simulink model "CryoDet"  (R2015b)
settings: Solver=ode45  SolverMode=SingleTasking  StartTime=0.0  StopTime=1e-4  MaxStep=1e-9  RelTol=1e-3
values from neighbouring files (symbols this model uses):
  Fclk = Fadc    (= 307200000)    [setupCryoFPGAxray.m]
  freqBusAddrBits = 4    [setupCryoFPGAxray.m]
  noise = exp(2i*pi*rand(1, noiseLen))    [setupCryoFPGAxray.m]
  noiseLen = 128    [setupCryoFPGAxray.m]
  noiseSteps = 32    [setupCryoFPGAxray.m]
  Tclk = 1/Fclk    (= 3.25520833333e-09)    [setupCryoFPGAxray.m]
undefined symbols (not defined in the file or in its folder): AXI4, Lite, notch, notch2, notch3, notch4, xlipgetpartsetting
libraries: xbsIndex_r4 x1227
(part 4 of 9)

== system CryoDet/DspCore/AdcDac 0/twelveLineUDC 0 ==
  In1 : Inport
  BDC scope : Scope  NumInputPorts=2
  Constant : xbsIndex_r4/Constant  const=0  gui_display_data_type=Fixed-point  arith_type=Unsigned  n_bits=4  bin_pt=0  preci_type=Single  exp_width=8  frac_width=24  explicit_period=off  period=1  equ=P=C  opselect=C  inp2=PCIN>>17  opr=+  inp1=P  carry=CIN  dbl_ovrd=off  block_type=constant
  Constant1 : xbsIndex_r4/Constant  const=1  gui_display_data_type=Fixed-point  arith_type=Unsigned  n_bits=4  bin_pt=0  preci_type=Single  exp_width=8  frac_width=24  explicit_period=off  period=1  equ=P=C  opselect=C  inp2=PCIN>>17  opr=+  inp1=P  carry=CIN  dbl_ovrd=off  block_type=constant
  Constant10 : xbsIndex_r4/Constant  const=10  gui_display_data_type=Fixed-point  arith_type=Unsigned  n_bits=4  bin_pt=0  preci_type=Single  exp_width=8  frac_width=24  explicit_period=off  period=1  equ=P=C  opselect=C  inp2=PCIN>>17  opr=+  inp1=P  carry=CIN  dbl_ovrd=off  block_type=constant
  Constant11 : xbsIndex_r4/Constant  const=11  gui_display_data_type=Fixed-point  arith_type=Unsigned  n_bits=4  bin_pt=0  preci_type=Single  exp_width=8  frac_width=24  explicit_period=off  period=1  equ=P=C  opselect=C  inp2=PCIN>>17  opr=+  inp1=P  carry=CIN  dbl_ovrd=off  block_type=constant
  Constant12 : xbsIndex_r4/Constant  const=15  gui_display_data_type=Fixed-point  arith_type=Unsigned  n_bits=4  bin_pt=0  preci_type=Single  exp_width=8  frac_width=24  explicit_period=off  period=1  equ=P=C  opselect=C  inp2=PCIN>>17  opr=+  inp1=P  carry=CIN  dbl_ovrd=off  block_type=constant
  Constant2 : xbsIndex_r4/Constant  const=2  gui_display_data_type=Fixed-point  arith_type=Unsigned  n_bits=4  bin_pt=0  preci_type=Single  exp_width=8  frac_width=24  explicit_period=off  period=1  equ=P=C  opselect=C  inp2=PCIN>>17  opr=+  inp1=P  carry=CIN  dbl_ovrd=off  block_type=constant
  Constant3 : xbsIndex_r4/Constant  const=3  gui_display_data_type=Fixed-point  arith_type=Unsigned  n_bits=4  bin_pt=0  preci_type=Single  exp_width=8  frac_width=24  explicit_period=off  period=1  equ=P=C  opselect=C  inp2=PCIN>>17  opr=+  inp1=P  carry=CIN  dbl_ovrd=off  block_type=constant
  Constant4 : xbsIndex_r4/Constant  const=4  gui_display_data_type=Fixed-point  arith_type=Unsigned  n_bits=4  bin_pt=0  preci_type=Single  exp_width=8  frac_width=24  explicit_period=off  period=1  equ=P=C  opselect=C  inp2=PCIN>>17  opr=+  inp1=P  carry=CIN  dbl_ovrd=off  block_type=constant
  Constant5 : xbsIndex_r4/Constant  const=5  gui_display_data_type=Fixed-point  arith_type=Unsigned  n_bits=4  bin_pt=0  preci_type=Single  exp_width=8  frac_width=24  explicit_period=off  period=1  equ=P=C  opselect=C  inp2=PCIN>>17  opr=+  inp1=P  carry=CIN  dbl_ovrd=off  block_type=constant
  Constant6 : xbsIndex_r4/Constant  const=6  gui_display_data_type=Fixed-point  arith_type=Unsigned  n_bits=4  bin_pt=0  preci_type=Single  exp_width=8  frac_width=24  explicit_period=off  period=1  equ=P=C  opselect=C  inp2=PCIN>>17  opr=+  inp1=P  carry=CIN  dbl_ovrd=off  block_type=constant
  Constant7 : xbsIndex_r4/Constant  const=7  gui_display_data_type=Fixed-point  arith_type=Unsigned  n_bits=4  bin_pt=0  preci_type=Single  exp_width=8  frac_width=24  explicit_period=off  period=1  equ=P=C  opselect=C  inp2=PCIN>>17  opr=+  inp1=P  carry=CIN  dbl_ovrd=off  block_type=constant
  Constant8 : xbsIndex_r4/Constant  const=8  gui_display_data_type=Fixed-point  arith_type=Unsigned  n_bits=4  bin_pt=0  preci_type=Single  exp_width=8  frac_width=24  explicit_period=off  period=1  equ=P=C  opselect=C  inp2=PCIN>>17  opr=+  inp1=P  carry=CIN  dbl_ovrd=off  block_type=constant
  Constant9 : xbsIndex_r4/Constant  const=9  gui_display_data_type=Fixed-point  arith_type=Unsigned  n_bits=4  bin_pt=0  preci_type=Single  exp_width=8  frac_width=24  explicit_period=off  period=1  equ=P=C  opselect=C  inp2=PCIN>>17  opr=+  inp1=P  carry=CIN  dbl_ovrd=off  block_type=constant
  Counter : xbsIndex_r4/Counter  cnt_type=Count Limited  cnt_to=15  operation=Up  start_count=0  cnt_by_val=1  arith_type=Unsigned  n_bits=4  bin_pt=0  load_pin=off  rst=on  en=on  explicit_period=off  period=Tclk  use_behavioral_HDL=off  implementation=Fabric  dbl_ovrd=off  block_type=counter
  DAC Sum : Subsystem
  Delay : xbsIndex_r4/Delay  rst=off  infoeditControl=Selection of Reset will increase slice count due to use of real FFs and instead of SRLs  en=off  latency=6  reg_retiming=off  dbl_ovrd=off  block_type=delay
  Demux : Demux
  Gateway Out{1,7..10,23} (6 alike) : xbsIndex_r4/Gateway Out  inherit_from_input=off  hdl_port=off  rows=1  columns=1  UseAsDAC=off  DACChannel='1'  interface=None  automatic_assignment=on  address_offset=hex2dec('00')  intf_name=''  intf_description=''  timing_constraint=None  locs_specified=off  LOCs={}  io_standard={}  block_type=gatewayout
  Mux12X4 : Subsystem
  Mux6 : Mux  Inputs=2
  Mux7 : Mux  Inputs=2
  Relational : xbsIndex_r4/Relational  mode=a!=b  op_type=Bool  en=off  latency=0  dbl_ovrd=off  block_type=relational
  SBdemod : Subsystem
  Toolbar : xbsIndex_r4/Toolbar  func=xltoolbar  block_type=toolbar
      settings: infoedit=Toolbar
  oneLineUpDown0 : Subsystem
  oneLineUpDown1 : Subsystem
  oneLineUpDown10 : Subsystem
  oneLineUpDown11 : Subsystem
  oneLineUpDown2 : Subsystem
  oneLineUpDown3 : Subsystem
  oneLineUpDown4 : Subsystem
  oneLineUpDown5 : Subsystem
  oneLineUpDown6 : Subsystem
  oneLineUpDown7 : Subsystem
  oneLineUpDown8 : Subsystem
  oneLineUpDown9 : Subsystem
  synch scope : Scope  NumInputPorts=2
  toDAC : Outport
  demodulated : Outport  Port=2
  wires:
  [fpgaReset] -> Counter/1, Delay/1
  oneLineUpDown7/1(Out1) -> Mux12X4/8(line7)
  oneLineUpDown6/1(Out1) -> Mux12X4/7(line6)
  oneLineUpDown5/1(Out1) -> Mux12X4/6(line5)
  oneLineUpDown4/1(Out1) -> Mux12X4/5(line4)
  oneLineUpDown3/1(Out1) -> Mux12X4/4(line3)
  oneLineUpDown2/1(Out1) -> Mux12X4/3(line2)
  Mux12X4/1(Out1) -> SBdemod/1(In1)
  oneLineUpDown1/1(Out1) -> Mux12X4/2(line1)
  oneLineUpDown0/1(Out1) -> Mux12X4/1(line0)
  oneLineUpDown8/1(Out1) -> Mux12X4/9(line8)
  oneLineUpDown9/1(Out1) -> Mux12X4/10(line9)
  oneLineUpDown10/1(Out1) -> Mux12X4/11(line10)
  oneLineUpDown11/1(Out1) -> Mux12X4/12(line11)
  oneLineUpDown11/2(toDAC) -> DAC Sum/12(In12)
  oneLineUpDown10/2(toDAC) -> DAC Sum/11(In11)
  oneLineUpDown9/2(toDAC) -> DAC Sum/10(In10)
  oneLineUpDown8/2(toDAC) -> DAC Sum/9(In9)
  oneLineUpDown7/2(toDAC) -> DAC Sum/8(In8)
  oneLineUpDown6/2(toDAC) -> DAC Sum/7(In7)
  oneLineUpDown5/2(toDAC) -> DAC Sum/6(In6)
  oneLineUpDown4/2(toDAC) -> DAC Sum/5(In5)
  oneLineUpDown3/2(toDAC) -> DAC Sum/4(In4)
  oneLineUpDown2/2(toDAC) -> DAC Sum/3(In3)
  oneLineUpDown1/2(toDAC) -> DAC Sum/2(In2)
  oneLineUpDown0/2(toDAC) -> DAC Sum/1(In1)
  DAC Sum/1(Out1) -> toDAC/1
  SBdemod/1(AllComponents) -> demodulated/1
  Gateway Out10/1 -> Mux7/2
  Gateway Out9/1 -> Mux7/1
  Gateway Out8/1 -> Mux6/2
  Gateway Out7/1 -> Mux6/1
  Mux6/1 -> BDC scope/1
  Mux7/1 -> BDC scope/2
  Demux/1 -> Gateway Out7/1
  Demux/4 -> Gateway Out10/1
  Demux/3 -> Gateway Out9/1
  Demux/2 -> Gateway Out8/1
  Delay/1 -> Mux12X4/13(synch)
  Constant/1 -> oneLineUpDown0/2(addrIn)
  Constant1/1 -> oneLineUpDown1/2(addrIn)
  Constant2/1 -> oneLineUpDown2/2(addrIn)
  Constant3/1 -> oneLineUpDown3/2(addrIn)
  Constant4/1 -> oneLineUpDown4/2(addrIn)
  Constant5/1 -> oneLineUpDown5/2(addrIn)
  Constant6/1 -> oneLineUpDown6/2(addrIn)
  Constant7/1 -> oneLineUpDown7/2(addrIn)
  Constant8/1 -> oneLineUpDown8/2(addrIn)
  Constant9/1 -> oneLineUpDown9/2(addrIn)
  Constant10/1 -> oneLineUpDown10/2(addrIn)
  Constant11/1 -> oneLineUpDown11/2(addrIn)
  In1/1 -> oneLineUpDown6/1(In), oneLineUpDown8/1(In), oneLineUpDown9/1(In), oneLineUpDown10/1(In), oneLineUpDown11/1(In), oneLineUpDown7/1(In), Demux/1, oneLineUpDown5/1(In), oneLineUpDown4/1(In), oneLineUpDown3/1(In), oneLineUpDown2/1(In), oneLineUpDown1/1(In), oneLineUpDown0/1(In)
  Counter/1 -> Gateway Out23/1, Relational/2, oneLineUpDown2/3(synchIn), oneLineUpDown3/3(synchIn), oneLineUpDown4/3(synchIn), oneLineUpDown5/3(synchIn), oneLineUpDown6/3(synchIn), oneLineUpDown7/3(synchIn), oneLineUpDown8/3(synchIn), oneLineUpDown10/3(synchIn), oneLineUpDown11/3(synchIn), oneLineUpDown9/3(synchIn), oneLineUpDown1/3(synchIn), oneLineUpDown0/3(synchIn)
  Gateway Out23/1 -> synch scope/1
  Gateway Out1/1 -> synch scope/2
  Relational/1 -> Gateway Out1/1, Counter/2
  Constant12/1 -> Relational/1

== system CryoDet/DspCore/AdcDac 0/twelveLineUDC 1 ==
  note: Null for now, eventually copy twelveLineUDC 0
      | when we need more than 12 lines per ADC channel
  In1 : Inport
  Out1 : Outport
  wires:
  In1/1 -> Out1/1

== system CryoDet/DspCore/AdcDac 0/LPF/CIC reset ==
  note: where N is number of channels in CIC filter
  note: reset latched resetIn
  note: latch resetIn
  note: CIC reset
      |
      | Synchronizes a CIC compiler 4.0 multi-channel CIC filter
      | to input channels
      |
      | Generates:
      | 1	notResetOut to CIC aresetn
      | 2	tlast to CIC tlast input
      |
      | Inputs:
      | 1	reset in
      | 2	Channel number (0-N) which may go to sel input of mux generating the input data stream
      | 3	N-2 which tells this module how deep is the multiplexing (e.g. N-2 = 10 for a 12 channel CIC filter (sorry))
      |
      | Guarantees:
      | 1	reset out is at least 2 clocks long
      | 2	end of reset occurs 2 clocks before channel 0
      | 3	tlast comes with channel N-1
      |
      | Assumes:
      | CIC oversampling set to "Sample period" = 1
      | No "streaming interface"
  resetIn : Inport
  Channel : Inport  Port=2
  N-2 : Inport  Port=3
  Constant : xbsIndex_r4/Constant  const=0  gui_display_data_type=Boolean  arith_type=Boolean  n_bits=16  bin_pt=14  preci_type=Single  exp_width=8  frac_width=24  explicit_period=off  period=1  equ=P=C  opselect=C  inp2=PCIN>>17  opr=+  inp1=P  carry=CIN  dbl_ovrd=off  block_type=constant
  Delay1 : xbsIndex_r4/Delay  rst=off  infoeditControl=Selection of Reset will increase slice count due to use of real FFs and instead of SRLs  en=off  latency=1  reg_retiming=off  dbl_ovrd=off  block_type=delay
  Delay2 : xbsIndex_r4/Delay  rst=off  infoeditControl=Selection of Reset will increase slice count due to use of real FFs and instead of SRLs  en=off  latency=1  reg_retiming=off  dbl_ovrd=off  block_type=delay
  Delay3 : xbsIndex_r4/Delay  rst=off  infoeditControl=Selection of Reset will increase slice count due to use of real FFs and instead of SRLs  en=off  latency=1  reg_retiming=off  dbl_ovrd=off  block_type=delay
  Inverter : xbsIndex_r4/Inverter  en=off  latency=2  dbl_ovrd=off  block_type=inv
  Inverter1 : xbsIndex_r4/Inverter  en=off  latency=0  dbl_ovrd=off  block_type=inv
  Logical : xbsIndex_r4/Logical  logical_function=AND  inputs=4  en=off  latency=0  precision=User Defined  arith_type=Boolean  n_bits=1  bin_pt=0  align_bp=on  dbl_ovrd=off  block_type=logical
  Logical1 : xbsIndex_r4/Logical  logical_function=OR  inputs=2  en=off  latency=0  precision=User Defined  arith_type=Boolean  n_bits=1  bin_pt=0  align_bp=on  dbl_ovrd=off  block_type=logical
  Mux : xbsIndex_r4/Mux  inputs=2  en=off  latency=0  precision=Full  arith_type=Unsigned  n_bits=16  bin_pt=14  quantization=Truncate  overflow=Wrap  dbl_ovrd=off  block_type=mux
  Relational1 : xbsIndex_r4/Relational  mode=a=b  op_type=Bool  en=off  latency=0  dbl_ovrd=off  block_type=relational
  notResetOut : Outport
  tlast : Outport  Port=2
  wires:
  resetIn/1 -> Inverter/1, Logical1/1
  Channel/1 -> Relational1/1
  N-2/1 -> Relational1/2
  Relational1/1 -> Logical/4, Delay1/1
  Logical1/1 -> Inverter1/1, Delay2/1
  Mux/1 -> Logical1/2
  Delay2/1 -> Logical/2, Delay3/1, Mux/2
  Constant/1 -> Mux/3
  Logical/1 -> Mux/1
  Delay1/1 -> tlast/1
  Inverter/1 -> Logical/1
  Delay3/1 -> Logical/3
  Inverter1/1 -> notResetOut/1

== system CryoDet/DspCore/AdcDac 0/SBmodulator/Phase Modulator ==
  Iin : Inport
  Qin : Inport  Port=2
  Ipm : Inport  Port=3
  Qpm : Inport  Port=4
  AddSub : xbsIndex_r4/AddSub  mode=Subtraction  use_carryin=off  use_carryout=off  en=off  latency=1  precision=User Defined  arith_type="Signed  (2's comp)"  n_bits=16  bin_pt=15  quantization=Truncate  overflow=Wrap  use_behavioral_HDL=off  hw_selection=Fabric  pipelined=off  dbl_ovrd=off  block_type=addsub
  AddSub1 : xbsIndex_r4/AddSub  mode=Addition  use_carryin=off  use_carryout=off  en=off  latency=1  precision=User Defined  arith_type="Signed  (2's comp)"  n_bits=16  bin_pt=15  quantization=Truncate  overflow=Wrap  use_behavioral_HDL=off  hw_selection=Fabric  pipelined=off  dbl_ovrd=off  block_type=addsub
  Mult{1..4} (4 alike) : xbsIndex_r4/Mult  precision=User Defined  arith_type="Signed  (2's comp)"  n_bits=16  bin_pt=15  quantization=Truncate  overflow=Wrap  en=off  latency=3  use_behavioral_HDL=off  opt=Speed  use_embedded=on  optimum_pipeline=off  pipeline=on  dbl_ovrd=off  use_rpm=on  placement_style=Triangular  block_type=mult
  Iout : Outport
  Qout : Outport  Port=2
  wires:
  Iin/1 -> Mult4/1, Mult2/1
  Qin/1 -> Mult1/1, Mult3/1
  Ipm/1 -> Mult2/2, Mult1/2
  Qpm/1 -> Mult3/2, Mult4/2
  Mult2/1 -> AddSub/1
  Mult3/1 -> AddSub/2
  Mult1/1 -> AddSub1/1
  Mult4/1 -> AddSub1/2
  AddSub/1 -> Iout/1
  AddSub1/1 -> Qout/1

== system CryoDet/DspCore/AdcDac 0/dF/CplxProd ==
  tvalidIn : Inport
  Im_A : Inport  Port=2
  Re_A : Inport  Port=3
  Im_B : Inport  Port=4
  Re_B : Inport  Port=5
  AddSub : xbsIndex_r4/AddSub  mode=Subtraction  use_carryin=off  use_carryout=off  en=off  latency=3  precision=Full  arith_type=Unsigned  n_bits=16  bin_pt=14  quantization=Truncate  overflow=Wrap  use_behavioral_HDL=off  hw_selection=DSP48  pipelined=on  dbl_ovrd=off  block_type=addsub
  AddSub1 : xbsIndex_r4/AddSub  mode=Addition  use_carryin=off  use_carryout=off  en=off  latency=3  precision=Full  arith_type=Unsigned  n_bits=16  bin_pt=14  quantization=Truncate  overflow=Wrap  use_behavioral_HDL=off  hw_selection=DSP48  pipelined=on  dbl_ovrd=off  block_type=addsub
  Delay : xbsIndex_r4/Delay  rst=off  infoeditControl=Selection of Reset will increase slice count due to use of real FFs and instead of SRLs  en=off  latency=3  reg_retiming=off  dbl_ovrd=off  block_type=delay
  Delay1 : xbsIndex_r4/Delay  rst=off  infoeditControl=Selection of Reset will increase slice count due to use of real FFs and instead of SRLs  en=off  latency=3  reg_retiming=off  dbl_ovrd=off  block_type=delay
  Mult{,1..3} (4 alike) : xbsIndex_r4/Mult  precision=Full  arith_type="Signed  (2's comp)"  n_bits=16  bin_pt=14  quantization=Truncate  overflow=Wrap  en=off  latency=3  use_behavioral_HDL=off  opt=Speed  use_embedded=on  optimum_pipeline=off  pipeline=on  dbl_ovrd=off  use_rpm=on  placement_style=Triangular  block_type=mult
  tvalidOut : Outport
  Im_Out : Outport  Port=2
  Re_Out : Outport  Port=3
  wires:
  Delay/1 -> Delay1/1
  Mult2/1 -> AddSub1/1
  Mult/1 -> AddSub/1
  Mult1/1 -> AddSub/2
  Mult3/1 -> AddSub1/2
  Re_A/1 -> Mult3/1, Mult/1
  Im_A/1 -> Mult2/1, Mult1/1
  tvalidIn/1 -> Delay/1
  Im_B/1 -> Mult1/2, Mult3/2
  Re_B/1 -> Mult/2, Mult2/2
  Delay1/1 -> tvalidOut/1
  AddSub/1 -> Re_Out/1
  AddSub1/1 -> Im_Out/1

== system CryoDet/DspCore/AdcDac 0/dF/CplxProd1 ==
  tvalidIn : Inport
  Im_A : Inport  Port=2
  Re_A : Inport  Port=3
  Im_B : Inport  Port=4
  Re_B : Inport  Port=5
  AddSub : xbsIndex_r4/AddSub  mode=Subtraction  use_carryin=off  use_carryout=off  en=off  latency=3  precision=Full  arith_type=Unsigned  n_bits=16  bin_pt=14  quantization=Truncate  overflow=Wrap  use_behavioral_HDL=off  hw_selection=DSP48  pipelined=on  dbl_ovrd=off  block_type=addsub
  AddSub1 : xbsIndex_r4/AddSub  mode=Addition  use_carryin=off  use_carryout=off  en=off  latency=3  precision=Full  arith_type=Unsigned  n_bits=16  bin_pt=14  quantization=Truncate  overflow=Wrap  use_behavioral_HDL=off  hw_selection=DSP48  pipelined=on  dbl_ovrd=off  block_type=addsub
  Delay : xbsIndex_r4/Delay  rst=off  infoeditControl=Selection of Reset will increase slice count due to use of real FFs and instead of SRLs  en=off  latency=3  reg_retiming=off  dbl_ovrd=off  block_type=delay
  Delay1 : xbsIndex_r4/Delay  rst=off  infoeditControl=Selection of Reset will increase slice count due to use of real FFs and instead of SRLs  en=off  latency=3  reg_retiming=off  dbl_ovrd=off  block_type=delay
  Mult{,1..3} (4 alike) : xbsIndex_r4/Mult  precision=Full  arith_type="Signed  (2's comp)"  n_bits=16  bin_pt=14  quantization=Truncate  overflow=Wrap  en=off  latency=3  use_behavioral_HDL=off  opt=Speed  use_embedded=on  optimum_pipeline=off  pipeline=on  dbl_ovrd=off  use_rpm=on  placement_style=Triangular  block_type=mult
  tvalidOut : Outport
  Im_Out : Outport  Port=2
  Re_Out : Outport  Port=3
  wires:
  Delay/1 -> Delay1/1
  Mult2/1 -> AddSub1/1
  Mult/1 -> AddSub/1
  Mult1/1 -> AddSub/2
  Mult3/1 -> AddSub1/2
  Re_A/1 -> Mult3/1, Mult/1
  Im_A/1 -> Mult2/1, Mult1/1
  tvalidIn/1 -> Delay/1
  Im_B/1 -> Mult1/2, Mult3/2
  Re_B/1 -> Mult/2, Mult2/2
  Delay1/1 -> tvalidOut/1
  AddSub/1 -> Re_Out/1
  AddSub1/1 -> Im_Out/1

== system CryoDet/DspCore/AdcDac 0/dF/dF lowpass ==
  note: Added integrator reset 23June2016
  note: If wTs not set, assume no filtering
  note: Channel repeats every 144 clocks
  note: IIR Lowpass filter
      | for frequency error
  chanIn : Inport
  "dFin " : Inport  Port=2
  AddSub2 : xbsIndex_r4/AddSub  mode=Addition  use_carryin=off  use_carryout=off  en=off  latency=4  precision=Full  arith_type="Signed  (2's comp)"  n_bits=24  bin_pt=16  quantization=Truncate  overflow=Saturate  use_behavioral_HDL=on  hw_selection=Fabric  pipelined=off  dbl_ovrd=off  block_type=addsub
  AddSub3 : xbsIndex_r4/AddSub  mode=Subtraction  use_carryin=off  use_carryout=off  en=off  latency=3  precision=Full  arith_type=Unsigned  n_bits=16  bin_pt=14  quantization=Truncate  overflow=Wrap  use_behavioral_HDL=off  hw_selection=Fabric  pipelined=off  dbl_ovrd=off  block_type=addsub
  Bus Creator : BusCreator  Inputs=2
  Bus Selector4 : BusSelector  OutputSignals=channel,freqError
  Constant : xbsIndex_r4/Constant  const=1  gui_display_data_type=Floating-point  arith_type=Floating-point  n_bits=16  bin_pt=14  preci_type=Single  exp_width=8  frac_width=24  explicit_period=off  period=1  equ=P=C  opselect=C  inp2=PCIN>>17  opr=+  inp1=P  carry=CIN  dbl_ovrd=off  block_type=constant
  Constant1 : xbsIndex_r4/Constant  const=0  gui_display_data_type=Floating-point  arith_type=Floating-point  n_bits=16  bin_pt=14  preci_type=Single  exp_width=8  frac_width=24  explicit_period=off  period=1  equ=P=C  opselect=C  inp2=PCIN>>17  opr=+  inp1=P  carry=CIN  dbl_ovrd=off  block_type=constant
  Constant5 : xbsIndex_r4/Constant  const=0  gui_display_data_type=Fixed-point  arith_type=Unsigned  n_bits=16  bin_pt=16  preci_type=Single  exp_width=8  frac_width=24  explicit_period=off  period=1  equ=P=C  opselect=C  inp2=PCIN>>17  opr=+  inp1=P  carry=CIN  dbl_ovrd=off  block_type=constant
  Constant6 : xbsIndex_r4/Constant  const=1  gui_display_data_type=Fixed-point  arith_type=Unsigned  n_bits=16  bin_pt=16  preci_type=Single  exp_width=8  frac_width=24  explicit_period=off  period=1  equ=P=C  opselect=C  inp2=PCIN>>17  opr=+  inp1=P  carry=CIN  dbl_ovrd=off  block_type=constant
  Convert : xbsIndex_r4/Convert  gui_display_data_type=Floating-point  arith_type=Floating-point  n_bits=16  bin_pt=14  float_type=Single  exp_bits=8  fraction_bits=24  quantization=Truncate  overflow=Wrap  en=off  latency=1  pipeline=off  dbl_ovrd=off  block_type=convert
  Convert1 : xbsIndex_r4/Convert  gui_display_data_type=Fixed-point  arith_type="Signed  (2's comp)"  n_bits=18  bin_pt=16  float_type=Single  exp_bits=8  fraction_bits=24  quantization=Truncate  overflow=Saturate  en=off  latency=1  pipeline=off  dbl_ovrd=off  block_type=convert
  Convert4 : xbsIndex_r4/Convert  gui_display_data_type=Fixed-point  arith_type="Signed  (2's comp)"  n_bits=32  bin_pt=30  float_type=Single  exp_bits=8  fraction_bits=24  quantization="Round  (unbiased: +/- Inf)"  overflow=Saturate  en=off  latency=1  pipeline=off  dbl_ovrd=off  block_type=convert
  Delay1 : xbsIndex_r4/Delay  rst=off  infoeditControl=Selection of Reset will increase slice count due to use of real FFs and instead of SRLs  en=off  latency=1  reg_retiming=off  dbl_ovrd=off  block_type=delay
  Delay2 : xbsIndex_r4/Delay  rst=off  infoeditControl=Selection of Reset will increase slice count due to use of real FFs and instead of SRLs  en=off  latency=3  reg_retiming=off  dbl_ovrd=off  block_type=delay
  Delay3 : xbsIndex_r4/Delay  rst=off  infoeditControl=Selection of Reset will increase slice count due to use of real FFs and instead of SRLs  en=off  latency=4  reg_retiming=off  dbl_ovrd=off  block_type=delay
  Display16 : Display
  Display17 : Display
  Gateway Out3 : xbsIndex_r4/Gateway Out  inherit_from_input=off  hdl_port=off  rows=1  columns=1  UseAsDAC=off  DACChannel='1'  interface=None  automatic_assignment=on  address_offset=hex2dec('00')  intf_name=''  intf_description=''  timing_constraint=None  locs_specified=off  LOCs={}  io_standard={}  block_type=gatewayout
  Gateway Out4 : xbsIndex_r4/Gateway Out  inherit_from_input=off  hdl_port=off  rows=1  columns=1  UseAsDAC=off  DACChannel='1'  interface=None  automatic_assignment=on  address_offset=hex2dec('00')  intf_name=''  intf_description=''  timing_constraint=None  locs_specified=off  LOCs={}  io_standard={}  block_type=gatewayout
  Mult2 : xbsIndex_r4/Mult  precision=Full  arith_type="Signed  (2's comp)"  n_bits=16  bin_pt=14  quantization=Truncate  overflow=Wrap  en=off  latency=3  use_behavioral_HDL=off  opt=Speed  use_embedded=on  optimum_pipeline=off  pipeline=on  dbl_ovrd=off  use_rpm=on  placement_style=Triangular  block_type=mult
  Mult3 : xbsIndex_r4/Mult  precision=Full  arith_type="Signed  (2's comp)"  n_bits=16  bin_pt=14  quantization=Truncate  overflow=Wrap  en=off  latency=140  use_behavioral_HDL=off  opt=Speed  use_embedded=on  optimum_pipeline=off  pipeline=on  dbl_ovrd=off  use_rpm=on  placement_style=Triangular  block_type=mult
  Mux1 : xbsIndex_r4/Mux  inputs=2  en=off  latency=0  precision=Full  arith_type=Unsigned  n_bits=16  bin_pt=14  quantization=Truncate  overflow=Wrap  dbl_ovrd=off  block_type=mux
  Mux3 : xbsIndex_r4/Mux  inputs=2  en=off  latency=1  precision=Full  arith_type=Unsigned  n_bits=16  bin_pt=14  quantization=Truncate  overflow=Wrap  dbl_ovrd=off  block_type=mux
  Relational2 : xbsIndex_r4/Relational  mode=a=b  op_type=Bool  en=off  latency=1  dbl_ovrd=off  block_type=relational
  dFLowpassscope : Scope  NumInputPorts=2
  Out1 : Outport
  wires:
  Bus Creator/1 -> Out1/1
  Constant/1 -> AddSub3/1
  Convert/1 -> Mult2/1, AddSub3/2
  Delay2/1 -> Delay3/1
  Convert1/1 -> Convert/1
  chanIn/1 -> Delay2/1
  Constant5/1 -> Relational2/1
  Relational2/1 -> Mux3/1
  Constant6/1 -> Mux3/3
  [omegaTsDf] -> Relational2/2, Mux3/2
  Mux3/1 -> Convert1/1
  Mult2/1 -> AddSub2/1
  "dFin "/1 -> Mult2/2
  Convert4/1 -> Bus Creator/2  "freqError"
  Delay1/1 -> Bus Creator/1  "channel"
  [dFbusLowPass] -> Bus Selector4/1
  Gateway Out4/1 -> Display17/1, dFLowpassscope/2
  Gateway Out3/1 -> dFLowpassscope/1, Display16/1
  Bus Selector4/1 -> Gateway Out3/1  "<channel>"
  Bus Selector4/2 -> Gateway Out4/1  "<freqError>"
  Mult3/1 -> AddSub2/2
  AddSub2/1 -> Mux1/2, Convert4/1
  Delay3/1 -> Delay1/1
  AddSub3/1 -> Mult3/2
  Mux1/1 -> Mult3/1
  [FBreset] -> Mux1/1
  Constant1/1 -> Mux1/3

== system CryoDet/DspCore/AdcDac 0/dF/etaRAM ==
  note: 4 May 2016 Now floating point
  readAddr : Inport
  "etaBusIn " : Inport  Port=2
  Bus Selector : BusSelector  OutputSignals=channel,etaQ,etaI
  Concat : xbsIndex_r4/Concat  num_inputs=2  dbl_ovrd=off  block_type=concat
  Dual Port RAM : xbsIndex_r4/Dual Port RAM  depth=2^freqBusAddrBits  initVector=0  distributed_mem=Block RAM  init_a=0  init_b=0  rst_a=off  rst_b=off  en_a=off  en_b=off  latency=2  write_mode_A=Read Before Write  write_mode_B=Read After Write  optimize=Area  dbl_ovrd=off  block_type=dpram
  Gateway Out{1..3,13,26,29} (6 alike) : xbsIndex_r4/Gateway Out  inherit_from_input=off  hdl_port=off  rows=1  columns=1  UseAsDAC=off  DACChannel='1'  interface=None  automatic_assignment=on  address_offset=hex2dec('00')  intf_name=''  intf_description=''  timing_constraint=None  locs_specified=off  LOCs={}  io_standard={}  block_type=gatewayout
  Mux1 : Mux  Inputs=2
  Mux13 : Mux  Inputs=2
  Mux7 : Mux  Inputs=2
  Reinterpret : xbsIndex_r4/Reinterpret  force_arith_type=on  arith_type=Unsigned  force_bin_pt=on  bin_pt=0  block_type=reinterpret
  Reinterpret1 : xbsIndex_r4/Reinterpret  force_arith_type=on  arith_type=Unsigned  force_bin_pt=on  bin_pt=0  block_type=reinterpret
  Reinterpret2 : xbsIndex_r4/Reinterpret  force_arith_type=on  arith_type=Floating-point  force_bin_pt=on  bin_pt=24  block_type=reinterpret
  Reinterpret3 : xbsIndex_r4/Reinterpret  force_arith_type=on  arith_type=Floating-point  force_bin_pt=on  bin_pt=24  block_type=reinterpret
  Slice : xbsIndex_r4/Slice  nbits=32  boolean_output=off  mode=Upper Bit Location + Width  bit1=0  base1=MSB of Input  bit0=0  base0=LSB of Input  dbl_ovrd=off  block_type=slice
  Slice1 : xbsIndex_r4/Slice  nbits=32  boolean_output=off  mode=Lower Bit Location + Width  bit1=0  base1=MSB of Input  bit0=0  base0=LSB of Input  dbl_ovrd=off  block_type=slice
  Terminator3 : Terminator
  eta ram in out : Scope  NumInputPorts=3
  read : xbsIndex_r4/Constant  const=0  gui_display_data_type=Boolean  arith_type=Boolean  n_bits=16  bin_pt=14  preci_type=Single  exp_width=8  frac_width=24  explicit_period=off  period=1  equ=P=C  opselect=C  inp2=PCIN>>17  opr=+  inp1=P  carry=CIN  dbl_ovrd=off  block_type=constant
  write : xbsIndex_r4/Constant  const=1.0  gui_display_data_type=Boolean  arith_type=Boolean  n_bits=16  bin_pt=14  preci_type=Single  exp_width=8  frac_width=24  explicit_period=off  period=1  equ=P=C  opselect=C  inp2=PCIN>>17  opr=+  inp1=P  carry=CIN  dbl_ovrd=off  block_type=constant
  etaQ : Outport
  etaI : Outport  Port=2
  wires:
  read/1 -> Dual Port RAM/6
  Bus Selector/1 -> Gateway Out26/1, Dual Port RAM/1  "<channel>"
  write/1 -> Dual Port RAM/3
  Dual Port RAM/2 -> Slice1/1, Slice/1
  Dual Port RAM/1 -> Terminator3/1
  "etaBusIn "/1 -> Bus Selector/1
  Bus Selector/2 -> Gateway Out2/1, Reinterpret/1  "<etaQ>"
  Bus Selector/3 -> Gateway Out29/1, Reinterpret1/1  "<etaI>"
  Reinterpret1/1 -> Concat/2
  Reinterpret/1 -> Concat/1
  Concat/1 -> Dual Port RAM/2, Dual Port RAM/5
  Slice/1 -> Reinterpret2/1
  Slice1/1 -> Reinterpret3/1
  Reinterpret2/1 -> Gateway Out1/1, etaQ/1
  Reinterpret3/1 -> Gateway Out3/1, etaI/1
  Gateway Out29/1 -> Mux13/1
  Mux13/1 -> eta ram in out/2
  Gateway Out13/1 -> Mux7/2
  Gateway Out26/1 -> Mux7/1
  Mux7/1 -> eta ram in out/1
  Gateway Out2/1 -> Mux13/2
  readAddr/1 -> Gateway Out13/1, Dual Port RAM/4
  Gateway Out3/1 -> Mux1/1
  Mux1/1 -> eta ram in out/3
  Gateway Out1/1 -> Mux1/2

== system CryoDet/DspCore/AdcDac 0/eta/Complex Divide ==
  note: Complex multiplier has latency 6
  a_tvalid : Inport
  A_Q : Inport  Port=2
  A_I : Inport  Port=3
  b_tvalid : Inport  Port=4
  B_Q : Inport  Port=5
  B_I : Inport  Port=6
  AddSub : xbsIndex_r4/AddSub  mode=Addition  use_carryin=off  use_carryout=off  en=off  latency=3  precision=Full  arith_type="Signed  (2's comp)"  n_bits=48  bin_pt=44  quantization=Truncate  overflow=Flag as error  use_behavioral_HDL=on  hw_selection=Fabric  pipelined=off  dbl_ovrd=off  block_type=addsub
  CMult : xbsIndex_r4/CMult  const=-1  gui_display_data_type=Floating-point  const_n_bits=16  const_bin_pt=15  float_type=Single  exp_bits=8  fraction_bits=24  en=off  latency=3  precision=Full  arith_type="Signed  (2's comp)"  n_bits=32  bin_pt=30  quantization=Truncate  overflow=Wrap  use_behavioral_HDL=off  mem_type=Distributed RAM  pipeline=off  dbl_ovrd=off  block_type=cmult
  Constant : xbsIndex_r4/Constant  const=0  gui_display_data_type=Floating-point  arith_type=Floating-point  n_bits=63  bin_pt=15  preci_type=Single  exp_width=8  frac_width=24  explicit_period=off  period=1  equ=P=C  opselect=C  inp2=PCIN>>17  opr=+  inp1=P  carry=CIN  dbl_ovrd=off  block_type=constant
  Cplx Div 2 : Scope  NumInputPorts=3
  CplxProd : Subsystem
  Cpx Div : Scope  NumInputPorts=4
  Delay{,1..2,5} (4 alike) : xbsIndex_r4/Delay  rst=off  infoeditControl=Selection of Reset will increase slice count due to use of real FFs and instead of SRLs  en=off  latency=3  reg_retiming=on  dbl_ovrd=off  block_type=delay
  Delay3 : xbsIndex_r4/Delay  rst=off  infoeditControl=Selection of Reset will increase slice count due to use of real FFs and instead of SRLs  en=off  latency=8  reg_retiming=on  dbl_ovrd=off  block_type=delay
  Divide : xbsIndex_r4/Divide  flow_control=NonBlocking  axi_optimize_goal=Resources  algorithm_type=Radix2  infoedit1=Specify output fraction-width for Fixed-point division.  fractional_width=24  infoedit2=Specify latency for Floating-point division.  latency=8  rate=1  has_a_tlast=off  has_a_tuser=off  has_b_tlast=off  has_b_tuser=off  en=off  has_result_tready=off  result_tlast_behv=Pass_A_TLAST  has_underflow=on  has_overflow=on  has_invalid_op=on  has_divide_by_zero=on  fpo_op_type=mergeddivide  block_type=divide
      settings: infoedit=Blocking: Wait for data on all inputs, allow back-pressure.<br>NonBlocking: operate every cycle in which all inputs are valid, no back-pressure.
  Divide1 : xbsIndex_r4/Divide  flow_control=NonBlocking  axi_optimize_goal=Resources  algorithm_type=Radix2  infoedit1=Specify output fraction-width for Fixed-point division.  fractional_width=24  infoedit2=Specify latency for Floating-point division.  latency=8  rate=1  has_a_tlast=off  has_a_tuser=off  has_b_tlast=off  has_b_tuser=off  en=off  has_result_tready=off  result_tlast_behv=Pass_A_TLAST  has_underflow=on  has_overflow=on  has_invalid_op=on  has_divide_by_zero=on  fpo_op_type=mergeddivide  block_type=divide
      settings: infoedit=Blocking: Wait for data on all inputs, allow back-pressure.<br>NonBlocking: operate every cycle in which all inputs are valid, no back-pressure.
  Gateway Out{1..2,6..17} (14 alike) : xbsIndex_r4/Gateway Out  inherit_from_input=off  hdl_port=off  rows=1  columns=1  UseAsDAC=off  DACChannel='1'  interface=None  automatic_assignment=on  address_offset=hex2dec('00')  intf_name=''  intf_description=''  timing_constraint=None  locs_specified=off  LOCs={}  io_standard={}  block_type=gatewayout
  Mult : xbsIndex_r4/Mult  precision=Full  arith_type="Signed  (2's comp)"  n_bits=48  bin_pt=44  quantization=Truncate  overflow=Flag as error  en=off  latency=6  use_behavioral_HDL=on  opt=Speed  use_embedded=on  optimum_pipeline=on  pipeline=on  dbl_ovrd=off  use_rpm=on  placement_style=Triangular  block_type=mult
  Mult1 : xbsIndex_r4/Mult  precision=Full  arith_type="Signed  (2's comp)"  n_bits=48  bin_pt=44  quantization=Truncate  overflow=Flag as error  en=off  latency=6  use_behavioral_HDL=on  opt=Speed  use_embedded=on  optimum_pipeline=off  pipeline=on  dbl_ovrd=off  use_rpm=on  placement_style=Triangular  block_type=mult
  Mux{1,3..5,8..10} (7 alike) : Mux  Inputs=2
  Mux6 : xbsIndex_r4/Mux  inputs=2  en=off  latency=0  precision=Full  arith_type=Unsigned  n_bits=63  bin_pt=15  quantization=Truncate  overflow=Flag as error  dbl_ovrd=off  block_type=mux
  Mux7 : xbsIndex_r4/Mux  inputs=2  en=off  latency=0  precision=Full  arith_type=Unsigned  n_bits=63  bin_pt=15  quantization=Truncate  overflow=Flag as error  dbl_ovrd=off  block_type=mux
  Terminator{,1..3,5} (5 alike) : Terminator
  Toolbar : xbsIndex_r4/Toolbar  func=xltoolbar  block_type=toolbar
      settings: infoedit=Toolbar
  tvalidOut : Outport
  Out_Q : Outport  Port=2
  Out_I : Outport  Port=3
  invalid op : Outport  Port=4
  wires:
  a_tvalid/1 -> Gateway Out13/1, Gateway Out12/1, Delay/1
  A_Q/1 -> Delay1/1, Gateway Out14/1
  A_I/1 -> Delay2/1, Gateway Out15/1
  Divide/1 -> Mux7/2
  Mult1/1 -> AddSub/2
  AddSub/1 -> Divide/2, Divide1/2
  Divide1/4 -> Gateway Out11/1, invalid op/1, Mux6/1, Mux7/1
  Mux7/1 -> Gateway Out6/1, Out_Q/1
  Mux6/1 -> Out_I/1, Gateway Out7/1
  Mult/1 -> AddSub/1
  Gateway Out6/1 -> Mux3/1
  Gateway Out7/1 -> Mux3/2
  Gateway Out8/1 -> Mux4/1
  Gateway Out9/1 -> Mux4/2
  Gateway Out10/1 -> Mux5/1
  Gateway Out11/1 -> Mux5/2
  Divide1/1 -> Mux6/2
  Constant/1 -> Mux7/3, Mux6/3
  Delay5/1 -> CplxProd/5(Re_B)
  Delay2/1 -> CplxProd/3(Re_A)
  Delay1/1 -> CplxProd/2(Im_A)
  Delay/1 -> CplxProd/1(tvalidIn)
  B_Q/1 -> Mult1/1, Mult1/2, Gateway Out16/1, CMult/1
  B_I/1 -> Mult/1, Mult/2, Delay5/1, Gateway Out17/1
  CMult/1 -> CplxProd/4(Im_B)
  Gateway Out12/1 -> Mux8/1
  Gateway Out13/1 -> Mux8/2
  Gateway Out14/1 -> Mux9/1
  Gateway Out15/1 -> Mux9/2
  Gateway Out16/1 -> Mux10/1
  Gateway Out17/1 -> Mux10/2
  Mux8/1 -> Cplx Div 2/1
  Mux9/1 -> Cplx Div 2/2
  Mux10/1 -> Cplx Div 2/3
  b_tvalid/1 -> Terminator5/1
  CplxProd/2(Im_Out) -> Divide/1
  CplxProd/1(tvalidOut) -> Gateway Out1/1, Delay3/1
  CplxProd/3(Re_Out) -> Divide1/1
  Divide1/2 -> Gateway Out8/1
  Divide1/3 -> Gateway Out9/1
  Divide1/5 -> Gateway Out10/1
  Mux3/1 -> Cpx Div/2
  Mux4/1 -> Cpx Div/3
  Mux5/1 -> Cpx Div/4
  Delay3/1 -> Gateway Out2/1, tvalidOut/1
  Mux1/1 -> Cpx Div/1
  Divide/2 -> Terminator/1
  Divide/3 -> Terminator1/1
  Divide/4 -> Terminator2/1
  Divide/5 -> Terminator3/1
  Gateway Out2/1 -> Mux1/2
  Gateway Out1/1 -> Mux1/1

== system CryoDet/DspCore/AdcDac 0/eta/CplxProd ==
  tvalidIn : Inport
  Im_A : Inport  Port=2
  Re_A : Inport  Port=3
  Im_B : Inport  Port=4
  Re_B : Inport  Port=5
  AddSub : xbsIndex_r4/AddSub  mode=Subtraction  use_carryin=off  use_carryout=off  en=off  latency=3  precision=Full  arith_type=Unsigned  n_bits=16  bin_pt=14  quantization=Truncate  overflow=Wrap  use_behavioral_HDL=off  hw_selection=DSP48  pipelined=on  dbl_ovrd=off  block_type=addsub
  AddSub1 : xbsIndex_r4/AddSub  mode=Addition  use_carryin=off  use_carryout=off  en=off  latency=3  precision=Full  arith_type=Unsigned  n_bits=16  bin_pt=14  quantization=Truncate  overflow=Wrap  use_behavioral_HDL=off  hw_selection=DSP48  pipelined=on  dbl_ovrd=off  block_type=addsub
  Delay : xbsIndex_r4/Delay  rst=off  infoeditControl=Selection of Reset will increase slice count due to use of real FFs and instead of SRLs  en=off  latency=3  reg_retiming=off  dbl_ovrd=off  block_type=delay
  Delay1 : xbsIndex_r4/Delay  rst=off  infoeditControl=Selection of Reset will increase slice count due to use of real FFs and instead of SRLs  en=off  latency=3  reg_retiming=off  dbl_ovrd=off  block_type=delay
  Mult{,1..3} (4 alike) : xbsIndex_r4/Mult  precision=Full  arith_type="Signed  (2's comp)"  n_bits=16  bin_pt=14  quantization=Truncate  overflow=Wrap  en=off  latency=3  use_behavioral_HDL=off  opt=Speed  use_embedded=on  optimum_pipeline=off  pipeline=on  dbl_ovrd=off  use_rpm=on  placement_style=Triangular  block_type=mult
  tvalidOut : Outport
  Im_Out : Outport  Port=2
  Re_Out : Outport  Port=3
  wires:
  Delay/1 -> Delay1/1
  Mult2/1 -> AddSub1/1
  Mult/1 -> AddSub/1
  Mult1/1 -> AddSub/2
  Mult3/1 -> AddSub1/2
  Re_A/1 -> Mult3/1, Mult/1
  Im_A/1 -> Mult2/1, Mult1/1
  tvalidIn/1 -> Delay/1
  Im_B/1 -> Mult1/2, Mult3/2
  Re_B/1 -> Mult/2, Mult2/2
  Delay1/1 -> tvalidOut/1
  AddSub/1 -> Re_Out/1
  AddSub1/1 -> Im_Out/1

== system CryoDet/DspCore/AdcDac 0/eta/CplxProd1 ==
  tvalidIn : Inport
  Im_A : Inport  Port=2
  Re_A : Inport  Port=3
  Im_B : Inport  Port=4
  Re_B : Inport  Port=5
  AddSub : xbsIndex_r4/AddSub  mode=Subtraction  use_carryin=off  use_carryout=off  en=off  latency=3  precision=Full  arith_type=Unsigned  n_bits=16  bin_pt=14  quantization=Truncate  overflow=Wrap  use_behavioral_HDL=off  hw_selection=DSP48  pipelined=on  dbl_ovrd=off  block_type=addsub
  AddSub1 : xbsIndex_r4/AddSub  mode=Addition  use_carryin=off  use_carryout=off  en=off  latency=3  precision=Full  arith_type=Unsigned  n_bits=16  bin_pt=14  quantization=Truncate  overflow=Wrap  use_behavioral_HDL=off  hw_selection=DSP48  pipelined=on  dbl_ovrd=off  block_type=addsub
  Delay : xbsIndex_r4/Delay  rst=off  infoeditControl=Selection of Reset will increase slice count due to use of real FFs and instead of SRLs  en=off  latency=3  reg_retiming=off  dbl_ovrd=off  block_type=delay
  Delay1 : xbsIndex_r4/Delay  rst=off  infoeditControl=Selection of Reset will increase slice count due to use of real FFs and instead of SRLs  en=off  latency=3  reg_retiming=off  dbl_ovrd=off  block_type=delay
  Mult{,1..3} (4 alike) : xbsIndex_r4/Mult  precision=Full  arith_type="Signed  (2's comp)"  n_bits=16  bin_pt=14  quantization=Truncate  overflow=Wrap  en=off  latency=3  use_behavioral_HDL=off  opt=Speed  use_embedded=on  optimum_pipeline=off  pipeline=on  dbl_ovrd=off  use_rpm=on  placement_style=Triangular  block_type=mult
  tvalidOut : Outport
  Im_Out : Outport  Port=2
  Re_Out : Outport  Port=3
  wires:
  Delay/1 -> Delay1/1
  Mult2/1 -> AddSub1/1
  Mult/1 -> AddSub/1
  Mult1/1 -> AddSub/2
  Mult3/1 -> AddSub1/2
  Re_A/1 -> Mult3/1, Mult/1
  Im_A/1 -> Mult2/1, Mult1/1
  tvalidIn/1 -> Delay/1
  Im_B/1 -> Mult1/2, Mult3/2
  Re_B/1 -> Mult/2, Mult2/2
  Delay1/1 -> tvalidOut/1
  AddSub/1 -> Re_Out/1
  AddSub1/1 -> Im_Out/1

== system CryoDet/DspCore/AdcDac 0/eta/CplxProd2 ==
  tvalidIn : Inport
  Im_A : Inport  Port=2
  Re_A : Inport  Port=3
  Im_B : Inport  Port=4
  Re_B : Inport  Port=5
  AddSub : xbsIndex_r4/AddSub  mode=Subtraction  use_carryin=off  use_carryout=off  en=off  latency=3  precision=Full  arith_type=Unsigned  n_bits=16  bin_pt=14  quantization=Truncate  overflow=Wrap  use_behavioral_HDL=off  hw_selection=DSP48  pipelined=on  dbl_ovrd=off  block_type=addsub
  AddSub1 : xbsIndex_r4/AddSub  mode=Addition  use_carryin=off  use_carryout=off  en=off  latency=3  precision=Full  arith_type=Unsigned  n_bits=16  bin_pt=14  quantization=Truncate  overflow=Wrap  use_behavioral_HDL=off  hw_selection=DSP48  pipelined=on  dbl_ovrd=off  block_type=addsub
  Delay : xbsIndex_r4/Delay  rst=off  infoeditControl=Selection of Reset will increase slice count due to use of real FFs and instead of SRLs  en=off  latency=3  reg_retiming=off  dbl_ovrd=off  block_type=delay
  Delay1 : xbsIndex_r4/Delay  rst=off  infoeditControl=Selection of Reset will increase slice count due to use of real FFs and instead of SRLs  en=off  latency=3  reg_retiming=off  dbl_ovrd=off  block_type=delay
  Mult{,1..3} (4 alike) : xbsIndex_r4/Mult  precision=Full  arith_type="Signed  (2's comp)"  n_bits=16  bin_pt=14  quantization=Truncate  overflow=Wrap  en=off  latency=3  use_behavioral_HDL=off  opt=Speed  use_embedded=on  optimum_pipeline=off  pipeline=on  dbl_ovrd=off  use_rpm=on  placement_style=Triangular  block_type=mult
  tvalidOut : Outport
  Im_Out : Outport  Port=2
  Re_Out : Outport  Port=3
  wires:
  Delay/1 -> Delay1/1
  Mult2/1 -> AddSub1/1
  Mult/1 -> AddSub/1
  Mult1/1 -> AddSub/2
  Mult3/1 -> AddSub1/2
  Re_A/1 -> Mult3/1, Mult/1
  Im_A/1 -> Mult2/1, Mult1/1
  tvalidIn/1 -> Delay/1
  Im_B/1 -> Mult1/2, Mult3/2
  Re_B/1 -> Mult/2, Mult2/2
  Delay1/1 -> tvalidOut/1
  AddSub/1 -> Re_Out/1
  AddSub1/1 -> Im_Out/1

== system CryoDet/DspCore/AdcDac 0/eta/IIR LPF ==
  note: Reasonably valid data ?
  chanIn : Inport
  Qin : Inport  Port=2
  Iin : Inport  Port=3
  inavalidIn : Inport  Port=4
  Absolute : xbsIndex_r4/Absolute  precision=Full  arith_type=Unsigned  n_bits=16  bin_pt=14  quantization=Truncate  overflow=Wrap  en=off  latency=1  dbl_ovrd=off  block_type=abs
  Absolute1 : xbsIndex_r4/Absolute  precision=Full  arith_type=Unsigned  n_bits=16  bin_pt=14  quantization=Truncate  overflow=Wrap  en=off  latency=1  dbl_ovrd=off  block_type=abs
  AddSub : xbsIndex_r4/AddSub  mode=Addition  use_carryin=off  use_carryout=off  en=off  latency=3  precision=Full  arith_type="Signed  (2's comp)"  n_bits=24  bin_pt=16  quantization=Truncate  overflow=Saturate  use_behavioral_HDL=on  hw_selection=Fabric  pipelined=off  dbl_ovrd=off  block_type=addsub
  AddSub1 : xbsIndex_r4/AddSub  mode=Subtraction  use_carryin=off  use_carryout=off  en=off  latency=3  precision=Full  arith_type=Unsigned  n_bits=16  bin_pt=14  quantization=Truncate  overflow=Wrap  use_behavioral_HDL=off  hw_selection=Fabric  pipelined=off  dbl_ovrd=off  block_type=addsub
  AddSub2 : xbsIndex_r4/AddSub  mode=Addition  use_carryin=off  use_carryout=off  en=off  latency=3  precision=Full  arith_type="Signed  (2's comp)"  n_bits=24  bin_pt=16  quantization=Truncate  overflow=Saturate  use_behavioral_HDL=on  hw_selection=Fabric  pipelined=off  dbl_ovrd=off  block_type=addsub
  AddSub3 : xbsIndex_r4/AddSub  mode=Addition  use_carryin=off  use_carryout=off  en=off  latency=3  precision=Full  arith_type=Unsigned  n_bits=16  bin_pt=14  quantization=Truncate  overflow=Wrap  use_behavioral_HDL=off  hw_selection=Fabric  pipelined=off  dbl_ovrd=off  block_type=addsub
  Complex to Magnitude-Angle : ComplexToMagnitudeAngle
  Complex to Magnitude-Angle1 : ComplexToMagnitudeAngle
  Constant : xbsIndex_r4/Constant  const=1  gui_display_data_type=Floating-point  arith_type=Floating-point  n_bits=16  bin_pt=14  preci_type=Single  exp_width=8  frac_width=24  explicit_period=off  period=1  equ=P=C  opselect=C  inp2=PCIN>>17  opr=+  inp1=P  carry=CIN  dbl_ovrd=off  block_type=constant
  Constant1 : xbsIndex_r4/Constant  const=1e5  gui_display_data_type=Floating-point  arith_type=Floating-point  n_bits=16  bin_pt=14  preci_type=Single  exp_width=8  frac_width=24  explicit_period=off  period=1  equ=P=C  opselect=C  inp2=PCIN>>17  opr=+  inp1=P  carry=CIN  dbl_ovrd=off  block_type=constant
  Constant2 : xbsIndex_r4/Constant  const=0  gui_display_data_type=Floating-point  arith_type=Floating-point  n_bits=16  bin_pt=14  preci_type=Single  exp_width=8  frac_width=24  explicit_period=off  period=1  equ=P=C  opselect=C  inp2=PCIN>>17  opr=+  inp1=P  carry=CIN  dbl_ovrd=off  block_type=constant
  Constant3 : xbsIndex_r4/Constant  const=0  gui_display_data_type=Fixed-point  arith_type=Unsigned  n_bits=16  bin_pt=16  preci_type=Single  exp_width=8  frac_width=24  explicit_period=off  period=1  equ=P=C  opselect=C  inp2=PCIN>>17  opr=+  inp1=P  carry=CIN  dbl_ovrd=off  block_type=constant
  Constant4 : xbsIndex_r4/Constant  const=1  gui_display_data_type=Fixed-point  arith_type=Unsigned  n_bits=16  bin_pt=16  preci_type=Single  exp_width=8  frac_width=24  explicit_period=off  period=1  equ=P=C  opselect=C  inp2=PCIN>>17  opr=+  inp1=P  carry=CIN  dbl_ovrd=off  block_type=constant
  Constant5 : xbsIndex_r4/Constant  const=0  gui_display_data_type=Floating-point  arith_type=Floating-point  n_bits=16  bin_pt=14  preci_type=Single  exp_width=8  frac_width=24  explicit_period=off  period=1  equ=P=C  opselect=C  inp2=PCIN>>17  opr=+  inp1=P  carry=CIN  dbl_ovrd=off  block_type=constant
  Convert : xbsIndex_r4/Convert  gui_display_data_type=Floating-point  arith_type=Floating-point  n_bits=16  bin_pt=14  float_type=Single  exp_bits=8  fraction_bits=24  quantization=Truncate  overflow=Wrap  en=off  latency=1  pipeline=off  dbl_ovrd=off  block_type=convert
  Convert1 : xbsIndex_r4/Convert  gui_display_data_type=Fixed-point  arith_type="Signed  (2's comp)"  n_bits=18  bin_pt=16  float_type=Single  exp_bits=8  fraction_bits=24  quantization=Truncate  overflow=Wrap  en=off  latency=1  pipeline=off  dbl_ovrd=off  block_type=convert
  Delay : xbsIndex_r4/Delay  rst=off  infoeditControl=Selection of Reset will increase slice count due to use of real FFs and instead of SRLs  en=off  latency=3  reg_retiming=off  dbl_ovrd=off  block_type=delay
  Delay1 : xbsIndex_r4/Delay  rst=off  infoeditControl=Selection of Reset will increase slice count due to use of real FFs and instead of SRLs  en=off  latency=3  reg_retiming=off  dbl_ovrd=off  block_type=delay
  Delay2 : xbsIndex_r4/Delay  rst=off  infoeditControl=Selection of Reset will increase slice count due to use of real FFs and instead of SRLs  en=off  latency=8  reg_retiming=off  dbl_ovrd=off  block_type=delay
  Delay3 : xbsIndex_r4/Delay  rst=off  infoeditControl=Selection of Reset will increase slice count due to use of real FFs and instead of SRLs  en=off  latency=8  reg_retiming=off  dbl_ovrd=off  block_type=delay
  Delay4 : xbsIndex_r4/Delay  rst=off  infoeditControl=Selection of Reset will increase slice count due to use of real FFs and instead of SRLs  en=off  latency=8  reg_retiming=off  dbl_ovrd=off  block_type=delay
  Display : Display
  Display1 : Display
  Gateway Out{,1..8} (9 alike) : xbsIndex_r4/Gateway Out  inherit_from_input=off  hdl_port=off  rows=1  columns=1  UseAsDAC=off  DACChannel='1'  interface=None  automatic_assignment=on  address_offset=hex2dec('00')  intf_name=''  intf_description=''  timing_constraint=None  locs_specified=off  LOCs={}  io_standard={}  block_type=gatewayout
  Logical : xbsIndex_r4/Logical  logical_function=AND  inputs=2  en=off  latency=1  precision=Full  arith_type=Unsigned  n_bits=16  bin_pt=0  align_bp=on  dbl_ovrd=off  block_type=logical
  Mult : xbsIndex_r4/Mult  precision=Full  arith_type="Signed  (2's comp)"  n_bits=16  bin_pt=14  quantization=Truncate  overflow=Wrap  en=off  latency=3  use_behavioral_HDL=off  opt=Speed  use_embedded=on  optimum_pipeline=off  pipeline=on  dbl_ovrd=off  use_rpm=on  placement_style=Triangular  block_type=mult
  Mult1 : xbsIndex_r4/Mult  precision=Full  arith_type="Signed  (2's comp)"  n_bits=16  bin_pt=14  quantization=Truncate  overflow=Wrap  en=off  latency="144*8 -  3"  use_behavioral_HDL=off  opt=Speed  use_embedded=on  optimum_pipeline=off  pipeline=on  dbl_ovrd=off  use_rpm=on  placement_style=Triangular  block_type=mult
  Mult2 : xbsIndex_r4/Mult  precision=Full  arith_type="Signed  (2's comp)"  n_bits=16  bin_pt=14  quantization=Truncate  overflow=Wrap  en=off  latency=3  use_behavioral_HDL=off  opt=Speed  use_embedded=on  optimum_pipeline=off  pipeline=on  dbl_ovrd=off  use_rpm=on  placement_style=Triangular  block_type=mult
  Mult3 : xbsIndex_r4/Mult  precision=Full  arith_type="Signed  (2's comp)"  n_bits=16  bin_pt=14  quantization=Truncate  overflow=Wrap  en=off  latency="144*8 -  3"  use_behavioral_HDL=off  opt=Speed  use_embedded=on  optimum_pipeline=off  pipeline=on  dbl_ovrd=off  use_rpm=on  placement_style=Triangular  block_type=mult
  Mux{,1,3..4} (4 alike) : xbsIndex_r4/Mux  inputs=2  en=off  latency=0  precision=Full  arith_type=Unsigned  n_bits=16  bin_pt=14  quantization=Truncate  overflow=Wrap  dbl_ovrd=off  block_type=mux
  Mux2 : xbsIndex_r4/Mux  inputs=2  en=off  latency=1  precision=Full  arith_type=Unsigned  n_bits=16  bin_pt=14  quantization=Truncate  overflow=Wrap  dbl_ovrd=off  block_type=mux
  Real-Imag to Complex : RealImagToComplex
  Real-Imag to Complex1 : RealImagToComplex
  Relational : xbsIndex_r4/Relational  mode=a<b  op_type=Bool  en=off  latency=3  dbl_ovrd=off  block_type=relational
  Relational1 : xbsIndex_r4/Relational  mode=a=b  op_type=Bool  en=off  latency=1  dbl_ovrd=off  block_type=relational
  eta lpf Scope : Scope  NumInputPorts=4
  eta lpf input qualifier : Scope  NumInputPorts=4
  mag eta in : Display
  mag eta out : Display
  chanOut : Outport
  Qout : Outport  Port=2
  Iout : Outport  Port=3
  wires:
  chanIn/1 -> Delay2/1
  Constant/1 -> AddSub1/1
  Convert/1 -> AddSub1/2, Gateway Out7/1, Mult2/1, Mult/1
  AddSub/1 -> Mux3/2, Mult/2
  Mult1/1 -> AddSub/2
  Qin/1 -> Absolute/1, Delay3/1
  AddSub1/1 -> Mult3/2, Mult1/2, Gateway Out8/1
  Mult/1 -> Gateway Out3/1, Qout/1
  Delay/1 -> Delay1/1
  Delay1/1 -> chanOut/1
  AddSub2/1 -> Mux4/2, Mult2/2
  Mult3/1 -> AddSub2/2
  Iin/1 -> Delay4/1, Absolute1/1
  Mult2/1 -> Gateway Out2/1, Iout/1
  Real-Imag to Complex/1 -> Complex to Magnitude-Angle/1
  Gateway Out1/1 -> Real-Imag to Complex/1
  Gateway Out/1 -> Real-Imag to Complex/2
  Real-Imag to Complex1/1 -> Complex to Magnitude-Angle1/1
  Gateway Out3/1 -> Real-Imag to Complex1/1
  Gateway Out2/1 -> Real-Imag to Complex1/2
  Complex to Magnitude-Angle/2 -> eta lpf Scope/4
  Complex to Magnitude-Angle/1 -> eta lpf input qualifier/1, mag eta in/1, eta lpf Scope/3
  Complex to Magnitude-Angle1/1 -> eta lpf Scope/1, mag eta out/1
  Complex to Magnitude-Angle1/2 -> eta lpf Scope/2
  Convert1/1 -> Convert/1
  Absolute1/1 -> AddSub3/1
  Absolute/1 -> AddSub3/2
  Relational/1 -> Logical/2
  AddSub3/1 -> Relational/2
  Constant1/1 -> Relational/1
  inavalidIn/1 -> Logical/1
  Mux/1 -> AddSub/1, Gateway Out1/1
  Logical/1 -> Gateway Out4/1, Mux1/1, Mux/1
  Mux1/1 -> Gateway Out/1, AddSub2/1
  Constant2/1 -> Mux1/3, Mux/3
  Delay2/1 -> Delay/1
  Delay3/1 -> Mux/2, Gateway Out6/1
  Delay4/1 -> Mux1/2, Gateway Out5/1
  Gateway Out4/1 -> eta lpf input qualifier/4
  Gateway Out5/1 -> eta lpf input qualifier/2
  Gateway Out6/1 -> eta lpf input qualifier/3
  Gateway Out8/1 -> Display/1
  Gateway Out7/1 -> Display1/1
  Constant3/1 -> Relational1/1
  Relational1/1 -> Mux2/1
  Constant4/1 -> Mux2/3
  [omegaTsPhiRef] -> Relational1/2, Mux2/2
  Mux2/1 -> Convert1/1
  Mux4/1 -> Mult3/1
  Mux3/1 -> Mult1/1
  [FBreset] -> Mux4/1, Mux3/1
  Constant5/1 -> Mux4/3, Mux3/3
